simulink model "roomtemp2"  (R2017b)
settings: Solver=ode45  StartTime=0.0  StopTime=86400  MaxStep=10  MinStep=0.00000001  RelTol=1e-6  AbsTol=1e-6  EnableMultiTasking=on
undefined symbols (not defined in the file or in its folder): Ca, Cw, Kf, Ki, Ko
libraries: simulink x4
settings Model: Creator=Andres  LastModifiedBy=Andres
settings DataIOCC: LimitDataPoints=on  SaveFormat=Array  SignalLoggingSaveFormat=ModelDataLogs  SaveOutput=off  SaveTime=off  SignalLoggingName=sigsOut
settings OptimizationCC: ExpressionDepthLimit=2147483647  InitFltsAndDblsToZero=on  LifeSpan=inf
settings DebuggingCC: SaveWithParameterizedLinksMsg=none  UnderspecifiedInitializationDetection=Classic  MergeDetectMultiDrivingBlocksExec=none  SignalResolutionControl=TryResolveAllWithWarning  MultiTaskDSMMsg=warning  MultiTaskCondExecSysMsg=none  FcnCallInpInsideContextMsg=warning  StateNameClashWarn=warning  StrictBusMsg=None  SFUnexpectedBacktrackingDiag=warning  SFNoUnconditionalDefaultTransitionDiag=warning  SFExecutionAtInitializationDiag=none
settings HardwareCC: ProdBitPerPointer=32  ProdBitPerSizeT=32  ProdBitPerPtrDiffT=32  ProdLargestAtomicFloat=None  ProdIntDivRoundTo=Undefined  ProdEndianess=Unspecified  ProdWordSize=32  ProdHWDeviceType=32-bit Generic  TargetUnknown=on
settings ModelReferenceCC: PropagateSignalLabelsOutOfModel=off
settings CodeAppCC: StateflowObjectComments=on
settings GRTTargetCC: TargetFcnLib=ansi_tfl_tmw.mat  TargetLangStandard=C89/C90 (ANSI)  CombineOutputUpdateFcns=off  GRTInterface=on
settings ConfigComp: CovMetricSettings=dw  CovHtmlReporting=on  CovSaveCumulativeToWorkspaceVar=on  CovSaveSingleToWorkspaceVar=on  CovExternalEMLEnable=off

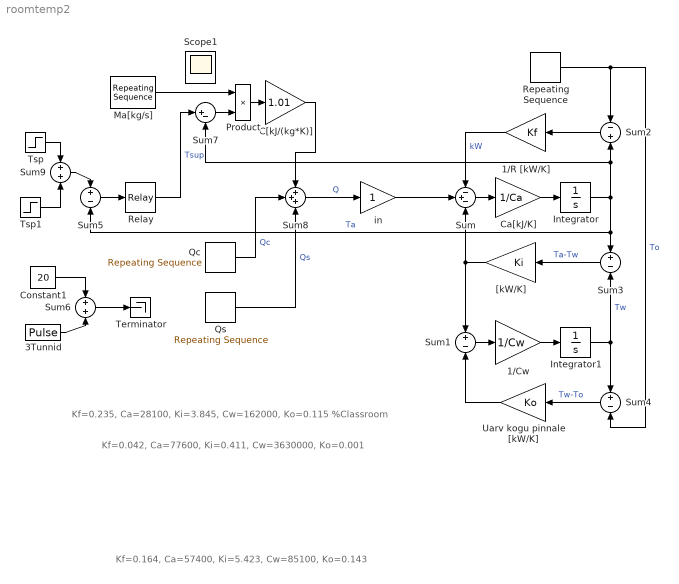
== system roomtemp2 ==
  note: Kf=0.235, Ca=28100, Ki=3.845, Cw=162000, Ko=0.115 %Classroom
  note: Kf=0.042, Ca=77600, Ki=0.411, Cw=3630000, Ko=0.001
  note: Kf=0.164, Ca=57400, Ki=5.423, Cw=85100, Ko=0.143
  1/Cw : Gain  Gain=1/Cw
  1/R [kW/K] : Gain  Gain=Kf
  3Tunnid : DiscretePulseGenerator  PulseType=Time based  Period=3600*3  PulseWidth=99
  C[kJ/(kg*K)] : Gain  Gain=1.01
  Ca[kJ/K] : Gain  Gain=1/Ca
  Constant1 : Constant  Value=20
  Integrator : Integrator  InitialCondition=20.5
  Integrator1 : Integrator  InitialCondition=20
  Ma[kg/s] : simulink/Sources/Repeating Sequence  rep_seq_t="[0  6.9 7  18.99  19 24] *3600"  rep_seq_y="[0  0 1  1  0   0]*0.75"
  Product : Product  RndMeth=Zero
  Qc : simulink/Sources/Repeating Sequence  rep_seq_t="[0  8 9  17  19 24] *3600"  rep_seq_y="[0  0 5  5  0   0]"
  Qs : simulink/Sources/Repeating Sequence  rep_seq_t="[0  9 11  16  17 24] *3600"  rep_seq_y="[0  0 0.2  0.2 0   0]*15.10"
  Relay : Relay  OnSwitchValue=0.5  OffSwitchValue=-0.5  OnOutputValue=21  OffOutputValue=18
  Repeating Sequence : simulink/Sources/Repeating Sequence  rep_seq_t="[0   7 12 16  20 24] *3600"  rep_seq_y="[10 9 13 13  10  8]"
  Sum : Sum  Inputs=-+-
  Sum{1,3..5} (4 alike) : Sum  Inputs=+-
  Sum2 : Sum  Inputs=-+
  Sum6 : Sum
  Sum7 : Sum  Inputs=|+-
  Sum8 : Sum  Inputs=+++
  Sum9 : Sum
  Terminator : Terminator
  Tsp : Step  Time=6*3600  Before=18  After=20.5  SampleTime=0
  Tsp1 : Step  Time=19*3600  After=-2.5  SampleTime=0
  Uarv kogu pinnale [kW/K] : Gain  Gain=Ko
  "[kW/K]" : Gain  Gain=Ki
  in : Gain
  Scope1 : Scope
  wires:
  Integrator/1 -> Sum3/1, Sum5/2, Sum2/2, Sum7/2  "Ta"
  "[kW/K]"/1 -> Sum1/1, Sum/3
  Sum1/1 -> 1/Cw/1
  Uarv kogu pinnale [kW/K]/1 -> Sum1/2
  Integrator1/1 -> Sum3/2, Sum4/1  "Tw"
  1/R [kW/K]/1 -> Sum/1  "kW"
  Ca[kJ/K]/1 -> Integrator/1
  1/Cw/1 -> Integrator1/1
  Sum2/1 -> 1/R [kW/K]/1
  Repeating Sequence/1 -> Sum4/2, Sum2/1  "To"
  Sum3/1 -> "[kW/K]"/1  "Ta-Tw"
  Sum4/1 -> Uarv kogu pinnale [kW/K]/1  "Tw-To"
  Relay/1 -> Sum7/1  "Tsup"
  Sum5/1 -> Relay/1
  Qc/1 -> Sum8/2  "Qc"
  Sum/1 -> Ca[kJ/K]/1
  Constant1/1 -> Sum6/1
  3Tunnid/1 -> Sum6/2
  Qs/1 -> Sum8/3  "Qs"
  Product/1 -> C[kJ/(kg*K)]/1
  C[kJ/(kg*K)]/1 -> Sum8/1
  Ma[kg/s]/1 -> Product/1
  Sum7/1 -> Product/2
  Sum8/1 -> in/1  "Q"
  in/1 -> Sum/2
  Tsp/1 -> Sum9/1
  Sum9/1 -> Sum5/1
  Tsp1/1 -> Sum9/2
  Sum6/1 -> Terminator/1
